simulink model "slot_machine"  (R2024b)
settings: Solver=VariableStepAuto  StartTime=0.0  StopTime=10000.0  RelTol=1e-3
model workspace (MAT data in the model file):
  hit = 1
libraries: dspswit3 x3
settings Model: Creator=anaca  LastModifiedBy=anaca

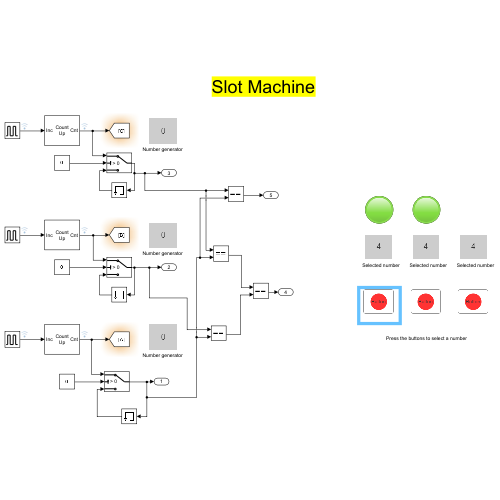
[thumbnail: Simulink's stored preview of the top-level diagram]
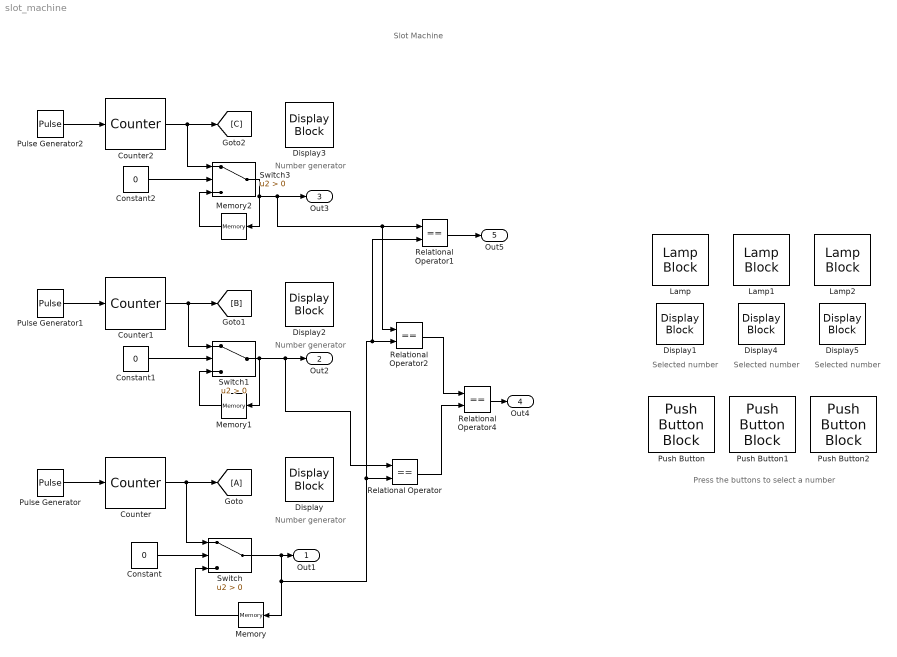
== system slot_machine ==
  note: Press the buttons to select a number
  note: Slot Machine
  note: Selected number
  note: Number generator
  note: Number generator
  note: Number generator
  note: Selected number
  note: Selected number
  Constant : Constant  Value=0
  Constant1 : Constant  Value=0
  Constant2 : Constant  Value=0
  Counter : dspswit3/Counter  Direction=Up  CountEvent=Rising edge  CounterSize=User defined  MaxCount=9  InitialCount=0  Output=Count  HitValue=hit  ResetInput=off  SamplesPerFrame=1  Ts=1  CntDtype=int8  HitDtype=Logical
  Counter1 : dspswit3/Counter  Direction=Up  CountEvent=Rising edge  CounterSize=User defined  MaxCount=9  InitialCount=0  Output=Count  HitValue=hit  ResetInput=off  SamplesPerFrame=1  Ts=1  CntDtype=int8  HitDtype=Logical
  Counter2 : dspswit3/Counter  Direction=Up  CountEvent=Rising edge  CounterSize=User defined  MaxCount=9  InitialCount=0  Output=Count  HitValue=hit  ResetInput=off  SamplesPerFrame=1  Ts=1  CntDtype=int8  HitDtype=Logical
  Display{,1..5} (6 alike) : DisplayBlock  LabelPosition=Hide  Transparency=1
  Goto : Goto
  Lamp : LampBlock  LabelPosition=Hide
  Lamp1 : LampBlock  LabelPosition=Hide
  Lamp2 : LampBlock  LabelPosition=Hide
  Memory : Memory
  Memory1 : Memory
  Memory2 : Memory
  Pulse Generator : DiscretePulseGenerator  PulseType=Time based  Period=0.0125
  Pulse Generator1 : DiscretePulseGenerator  PulseType=Time based  Period=0.0200  PulseWidth=0.3
  Pulse Generator2 : DiscretePulseGenerator  PulseType=Time based  Period=0.04  PulseWidth=0.1
  Push Button : PushButtonBlock  Icon=Circle  CustomIcon=data:image/png;base64,/9j/4AAQSkZJRgABAQAAAQABAAD/2wBDAAEBAQEBAQEBAQEBAQEBAQEBAQEBAQEBAQEBAQEBAQEBAQEBAQEBAQEBAQEBAQEBAQEBAQEBAQEBAQEBAQEBAQH/2wBDAQEBAQEBAQEBAQEBAQEBAQEBAQEBAQEBAQEBAQEBAQEBAQEBAQEBAQEBAQEBAQEBAQEBAQEBAQEBAQEBAQEBAQH/wAARCANrA0gDASIAAhEBAxEB/8QAHwAAAQUBAQEBAQEAAAAAAAAAAAECAwQFBgcICQoL/8QAtRAAAgEDAwIEAwUFBAQAAAF9AQIDAAQRBRIhMUEGE1FhByJxFDKBkaEII0KxwRVS0fAkM2JyggkKFhcYGRolJicoKSo0NTY3ODk6Q0RFRkdISUpTVFVW ...(+228192 chars)  IconAlignment=Center  IconColor=On  OffValue=0.000000
  Push Button1 : PushButtonBlock  Icon=Circle  CustomIcon=data:image/png;base64,/9j/4AAQSkZJRgABAQAAAQABAAD/2wBDAAEBAQEBAQEBAQEBAQEBAQEBAQEBAQEBAQEBAQEBAQEBAQEBAQEBAQEBAQEBAQEBAQEBAQEBAQEBAQEBAQEBAQH/2wBDAQEBAQEBAQEBAQEBAQEBAQEBAQEBAQEBAQEBAQEBAQEBAQEBAQEBAQEBAQEBAQEBAQEBAQEBAQEBAQEBAQEBAQH/wAARCANrA0gDASIAAhEBAxEB/8QAHwAAAQUBAQEBAQEAAAAAAAAAAAECAwQFBgcICQoL/8QAtRAAAgEDAwIEAwUFBAQAAAF9AQIDAAQRBRIhMUEGE1FhByJxFDKBkaEII0KxwRVS0fAkM2JyggkKFhcYGRolJicoKSo0NTY3ODk6Q0RFRkdISUpTVFVW ...(+228192 chars)  IconAlignment=Center  IconColor=On  OffValue=0.000000
  Push Button2 : PushButtonBlock  Icon=Circle  CustomIcon=data:image/png;base64,/9j/4AAQSkZJRgABAQAAAQABAAD/2wBDAAEBAQEBAQEBAQEBAQEBAQEBAQEBAQEBAQEBAQEBAQEBAQEBAQEBAQEBAQEBAQEBAQEBAQEBAQEBAQEBAQEBAQH/2wBDAQEBAQEBAQEBAQEBAQEBAQEBAQEBAQEBAQEBAQEBAQEBAQEBAQEBAQEBAQEBAQEBAQEBAQEBAQEBAQEBAQEBAQH/wAARCANrA0gDASIAAhEBAxEB/8QAHwAAAQUBAQEBAQEAAAAAAAAAAAECAwQFBgcICQoL/8QAtRAAAgEDAwIEAwUFBAQAAAF9AQIDAAQRBRIhMUEGE1FhByJxFDKBkaEII0KxwRVS0fAkM2JyggkKFhcYGRolJicoKSo0NTY3ODk6Q0RFRkdISUpTVFVW ...(+228192 chars)  IconAlignment=Center  IconColor=On  OffValue=0.000000
  Relational Operator{,1..2,4} (4 alike) : RelationalOperator  Operator===  OutDataTypeStr=boolean  RndMeth=Simplest  InputSameDT=off
  Switch : Switch  Criteria=u2 > Threshold  SaturateOnIntegerOverflow=off  InputSameDT=off
  Switch1 : Switch  Criteria=u2 > Threshold  SaturateOnIntegerOverflow=off  InputSameDT=off
  Switch3 : Switch  Criteria=u2 > Threshold  SaturateOnIntegerOverflow=off  InputSameDT=off
  Out1 : Outport
  Out2 : Outport  Port=2
  Out3 : Outport  Port=3
  Out4 : Outport  Port=4
  Out5 : Outport  Port=5
  wires:
  Pulse Generator/1 -> Counter/1
  Counter/1 -> Switch/1, Goto/1
  Constant/1 -> Switch/2
  Switch/1 -> Out1/1, Memory/1, Relational Operator2/2, Relational Operator1/2, Relational Operator/2
  Memory/1 -> Switch/3
  Counter1/1 -> Switch1/1, [B]
  Counter2/1 -> Switch3/1, [C]
  Pulse Generator1/1 -> Counter1/1
  Pulse Generator2/1 -> Counter2/1
  Switch1/1 -> Relational Operator/1, Out2/1, Memory1/1
  Memory1/1 -> Switch1/3
  Switch3/1 -> Relational Operator2/1, Relational Operator1/1, Out3/1, Memory2/1
  Memory2/1 -> Switch3/3
  Constant1/1 -> Switch1/2
  Constant2/1 -> Switch3/2
  Relational Operator2/1 -> Relational Operator4/1
  Relational Operator/1 -> Relational Operator4/2
  Relational Operator4/1 -> Out4/1
  Relational Operator1/1 -> Out5/1
